simulink model "ELECTRIC_RC_AIRCRAFT_backup_1"  (R2025b)
settings: Solver=VariableStepAuto  StartTime=0.0  StopTime=60  RelTol=1e-3
values from neighbouring files (symbols this model uses):
  g = 9.81    [ELECTRIC_RC_AIRCRAFT.m]
  m = 1.83    [ELECTRIC_RC_AIRCRAFT.m]
libraries: aerolibadyn x1, aerolibatmos2 x1, aerolibasang x1, aerolibbdyn x1, aerolibpropulsion2 x1
settings Model: Creator=papar  LastModifiedBy=papar

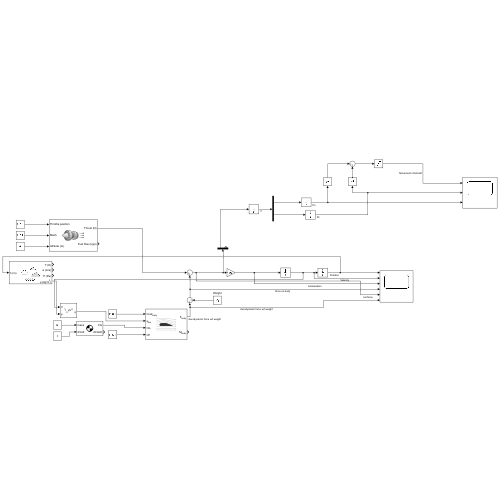
[thumbnail: Simulink's stored preview of the top-level diagram]
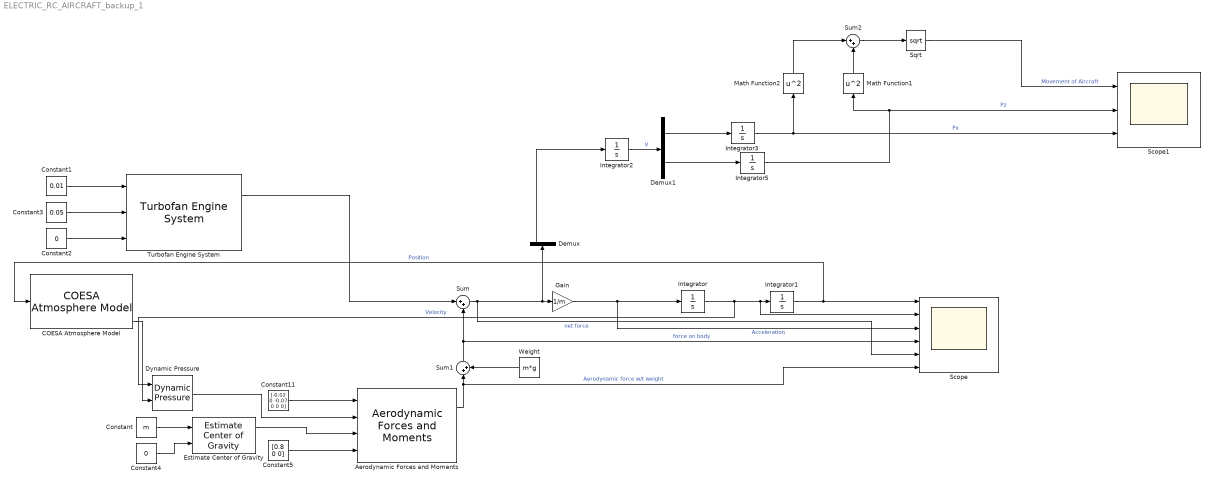
== system ELECTRIC_RC_AIRCRAFT_backup_1 ==
  "Aerodynamic Forces and Moments " : aerolibadyn/Aerodynamic Forces and Moments   inputAxes=Body  outputForceAxes=Body  outputMomentAxes=Body  S=1.67  b=3.66  cbar=2.13
  COESA Atmosphere Model : aerolibatmos2/COESA Atmosphere Model  units=Metric (MKS)  spec=1976 COESA-extended U.S. Standard Atmosphere  model=Profile  profile_var=High temperature  profile_percent=1%  profile_alt=5 km (16404 ft)  envelope_var=High temperature  envelope_percent=1%  action=Warning
  Constant : Constant  Value=m
  Constant1 : Constant  Value=0.01
  Constant11 : Constant  Value=[-0.02 0 -0.07 0 0 0]
  Constant2 : Constant  Value=0
  Constant3 : Constant  Value=0.05
  Constant4 : Constant  Value=0
  Constant5 : Constant  Value=[0.8 0 0]
  Demux : Demux  Outputs=2
  Demux1 : Demux  Outputs=2
  Dynamic Pressure : aerolibasang/Dynamic Pressure
  Estimate Center of Gravity : aerolibbdyn/Estimate Center of Gravity  fmass=m  emass=m  fcg=[0 0 0]'  ecg=[0 0 0]'
  Gain : Gain  Gain=1/m
  Integrator : Integrator  ContinuousStateAttributes='Velocity'
  Integrator1 : Integrator
  Integrator2 : Integrator  ContinuousStateAttributes='Velocity'
  Integrator3 : Integrator
  Integrator5 : Integrator
  Math Function1 : Math  Operator=square
  Math Function2 : Math  Operator=square
  Scope : Scope  NumInputPorts=6
      settings: TimeDisplayOffset=1  ActiveDisplayYMinimum=-2657.0869830977408  ActiveDisplayYMaximum=1787.4090222471134  DataLoggingMaxPoints=500
  Scope1 : Scope  NumInputPorts=3
      settings: ActiveDisplayYMinimum=-17677.925333115367  ActiveDisplayYMaximum=85692.487742886515
  Sqrt : Sqrt
  Sum : Sum  Inputs=|++
  Sum1 : Sum  Inputs=|++
  Sum2 : Sum  Inputs=|++
  Turbofan Engine System : aerolibpropulsion2/Turbofan Engine System  units=Metric (MKS)  ic_source=Internal  IC=0  Fmax=20  tau=0.4  SFC=0  Nt=0.9
  Weight : Constant  Value=m*g
  wires:
  Integrator/1 -> Dynamic Pressure/1, Scope/2, Integrator1/1  "Velocity"
  Integrator1/1 -> COESA Atmosphere Model/1, Scope/1  "Position"
  Gain/1 -> Integrator/1, Scope/3  "Acceleration"
  Constant1/1 -> Turbofan Engine System/1
  Constant2/1 -> Turbofan Engine System/3
  Constant3/1 -> Turbofan Engine System/2
  Dynamic Pressure/1 -> "Aerodynamic Forces and Moments "/2
  Estimate Center of Gravity/1 -> "Aerodynamic Forces and Moments "/3
  Turbofan Engine System/1 -> Sum/1
  Sum/1 -> Demux/1, Gain/1, Scope/5  "net force"
  Constant/1 -> Estimate Center of Gravity/1
  Constant4/1 -> Estimate Center of Gravity/2
  Constant11/1 -> "Aerodynamic Forces and Moments "/1
  Constant5/1 -> "Aerodynamic Forces and Moments "/4
  COESA Atmosphere Model/4 -> Dynamic Pressure/2
  "Aerodynamic Forces and Moments "/1 -> Scope/6, Sum1/1  "Aerodynamic force w/t weight"
  Sum1/1 -> Sum/2, Scope/4  "force on body"
  Weight/1 -> Sum1/2
  Demux/1 -> Integrator2/1
  Integrator2/1 -> Demux1/1  "V"
  Demux1/2 -> Integrator5/1
  Demux1/1 -> Integrator3/1
  Integrator5/1 -> Math Function1/1, Scope1/2  "Pz"
  Integrator3/1 -> Math Function2/1, Scope1/3  "Px"
  Math Function2/1 -> Sum2/1
  Math Function1/1 -> Sum2/2
  Sum2/1 -> Sqrt/1
  Sqrt/1 -> Scope1/1  "Movement of Aircraft"
